simulink model "GolfSwingLogging"  (R2024b)
settings: Solver=VariableStepAuto  StartTime=0.0  StopTime=StopTime  MaxStep=0.001  RelTol=1e-3
PreLoadFcn:
  | cd(matlabdrive);
  | cd '2DModel';
PostLoadFcn:
  | %run SCRIPT_mdlWksGenerate.m;
  | mdlWks=get_param('GolfSwing','ModelWorkspace');
  | mdlWks.DataSource = 'MAT-File';
  | mdlWks.FileName = 'ModelInputs.mat';
  | mdlWks.reload;
model workspace: external: MAT-File ModelInputs.mat (data not in the file)
undefined symbols (not defined in the file or in its folder): GlobalGain, HipConstant, HipDampening, HipTimeGain, KillDampFinalValue, KillDampInitialValue, KillswitchFinalValue, KillswitchInitialValue, KillswitchStepTime, LElbowConstant, LElbowDampening, LElbowTimeGain, LScapConstant, LScapDampening, LScapPositionGain, LScapTimeGain, LShoulderConstant, LShoulderDampening, LShoulderTimeGain, LWristConstant, LWristDampening, LWristTimeGain, RElbowConstant, RElbowDampening, RElbowTimeGain, RScapConstant, RScapDampening, RScapPositionGain, RScapTimeGain, RShoulderConstant, RShoulderDampening, RShoulderTimeGain, RWristConstant, RWristDampening, RWristTimeGain, TorsoConstant, TorsoDampening, TorsoPositionGain, TorsoTimeGain, WristGain, X, Y, Z
libraries: nesl_utility x204, sm_lib x102, matrix_library x11, simulink_extras x2, simulink x1
(part 5 of 6)

== system GolfSwingLogging/Club/ButtGlobal ==
  Buttx : nesl_utility/PS-Simulink Converter  PhysicalDomain=network_engine_domain  SubClassName=ps_output  LeftPortType=input  RightPortType=output  PseudoPeriodic=off  Frequencies=[]  VectorFormat=1-D array  Unit=inherit  AffineConversion=off
  Butty : nesl_utility/PS-Simulink Converter  PhysicalDomain=network_engine_domain  SubClassName=ps_output  LeftPortType=input  RightPortType=output  PseudoPeriodic=off  Frequencies=[]  VectorFormat=1-D array  Unit=inherit  AffineConversion=off
  Buttz : nesl_utility/PS-Simulink Converter  PhysicalDomain=network_engine_domain  SubClassName=ps_output  LeftPortType=input  RightPortType=output  PseudoPeriodic=off  Frequencies=[]  VectorFormat=1-D array  Unit=inherit  AffineConversion=off
  Transform Sensor : sm_lib/Frames and Transforms/Transform Sensor  MeasurementFrame=World  RotationSequence=XYX  SenseAngle=off  SenseAxis=off  SenseQ=off  SenseR=off  SenseRotationSequence=off  SenseOmegaX=off  SenseOmegaY=off  SenseOmegaZ=off  SenseOmega=off  SenseQDot=off  SenseRDot=off  SenseRotationSequenceDot=off  SenseAlphaX=off  SenseAlphaY=off  SenseAlphaZ=off  SenseAlpha=off  SenseQDDot=off  SenseRDDot=off  SenseX=on  SenseY=on  SenseZ=on  SenseXYZ=off  SenseRad=off  SenseAzim=off  SenseDist=off  SenseInc=off  SenseXDot=off  SenseYDot=off  SenseZDot=off  SenseXYZDot=off  SenseRadDot=off  SenseAzimDot=off  SenseDistDot=off  SenseIncDot=off  SenseXDDot=off  SenseYDDot=off  SenseZDDot=off  SenseXYZDDot=off  SenseRadDDot=off  SenseAzimDDot=off  SenseDistDDot=off  SenseIncDDot=off
  Conn1 : PMIOPort  Side=Right
  Conn2 : PMIOPort  Port=2  Side=Left
  connections:
  Buttx/LConn1 -- Transform Sensor/RConn2
  Buttz/LConn1 -- Transform Sensor/RConn4
  Butty/LConn1 -- Transform Sensor/RConn3
  Transform Sensor/LConn1 -- Conn2/RConn1
  Transform Sensor/RConn1 -- Conn1/RConn1

== system GolfSwingLogging/Club/CHGlobal ==
  AoA Calculation : Subsystem
  CHS (m/s) : Subsystem
  CHSmph : Gain  Gain=2.23694
  CHvx : nesl_utility/PS-Simulink Converter  PhysicalDomain=network_engine_domain  SubClassName=ps_output  LeftPortType=input  RightPortType=output  PseudoPeriodic=off  Frequencies=[]  VectorFormat=1-D array  Unit=inherit  AffineConversion=off
  CHvy : nesl_utility/PS-Simulink Converter  PhysicalDomain=network_engine_domain  SubClassName=ps_output  LeftPortType=input  RightPortType=output  PseudoPeriodic=off  Frequencies=[]  VectorFormat=1-D array  Unit=inherit  AffineConversion=off
  CHvz : nesl_utility/PS-Simulink Converter  PhysicalDomain=network_engine_domain  SubClassName=ps_output  LeftPortType=input  RightPortType=output  PseudoPeriodic=off  Frequencies=[]  VectorFormat=1-D array  Unit=inherit  AffineConversion=off
  CHx : nesl_utility/PS-Simulink Converter  PhysicalDomain=network_engine_domain  SubClassName=ps_output  LeftPortType=input  RightPortType=output  PseudoPeriodic=off  Frequencies=[]  VectorFormat=1-D array  Unit=inherit  AffineConversion=off
  CHy : nesl_utility/PS-Simulink Converter  PhysicalDomain=network_engine_domain  SubClassName=ps_output  LeftPortType=input  RightPortType=output  PseudoPeriodic=off  Frequencies=[]  VectorFormat=1-D array  Unit=inherit  AffineConversion=off
  CHz : nesl_utility/PS-Simulink Converter  PhysicalDomain=network_engine_domain  SubClassName=ps_output  LeftPortType=input  RightPortType=output  PseudoPeriodic=off  Frequencies=[]  VectorFormat=1-D array  Unit=inherit  AffineConversion=off
  ClubheadPathUnitVector : Mux  Inputs=3
  Constant : Constant  Value=0
  Filtering Block : Subsystem  Commented=on
  MinMax Running Resettable : simulink/Math Operations/MinMax Running Resettable  Function=max  vinit=0.0
  Path Calculation : Subsystem
  Transform Sensor : sm_lib/Frames and Transforms/Transform Sensor  MeasurementFrame=World  RotationSequence=XYX  SenseAngle=off  SenseAxis=off  SenseQ=off  SenseR=off  SenseRotationSequence=off  SenseOmegaX=off  SenseOmegaY=off  SenseOmegaZ=off  SenseOmega=off  SenseQDot=off  SenseRDot=off  SenseRotationSequenceDot=off  SenseAlphaX=off  SenseAlphaY=off  SenseAlphaZ=off  SenseAlpha=off  SenseQDDot=off  SenseRDDot=off  SenseX=on  SenseY=on  SenseZ=on  SenseXYZ=off  SenseRad=off  SenseAzim=off  SenseDist=off  SenseInc=off  SenseXDot=on  SenseYDot=on  SenseZDot=on  SenseXYZDot=off  SenseRadDot=off  SenseAzimDot=off  SenseDistDot=off  SenseIncDot=off  SenseXDDot=off  SenseYDDot=off  SenseZDDot=off  SenseXYZDDot=off  SenseRadDDot=off  SenseAzimDDot=off  SenseDistDDot=off  SenseIncDDot=off
  UnitVectorX : Product  Inputs=*/
  UnitVectorY : Product  Inputs=*/
  UnitVectorZ : Product  Inputs=*/
  Clubhead : PMIOPort  Side=Right
  Global : PMIOPort  Port=2  Side=Left
  ClubPathUV : Outport
  CHSMPS : Outport  Port=2
  wires:
  CHvy/1 -> Path Calculation/1(Vy), AoA Calculation/2(Vy), UnitVectorY/1, CHS (m/s)/2(In2)  "CHvy"
  CHvx/1 -> AoA Calculation/1(Vx), Path Calculation/2(Vx), UnitVectorX/1, CHS (m/s)/1(In1)  "CHvx"
  CHvz/1 -> CHS (m/s)/3(In3), AoA Calculation/3(Vz), UnitVectorZ/1  "CHvz"
  UnitVectorZ/1 -> ClubheadPathUnitVector/3
  UnitVectorY/1 -> ClubheadPathUnitVector/2
  CHS (m/s)/1(ClubPathUV1) -> CHSMPS/1, CHSmph/1, UnitVectorZ/2, UnitVectorY/2, UnitVectorX/2  "CHSmpersec"
  UnitVectorX/1 -> ClubheadPathUnitVector/1
  ClubheadPathUnitVector/1 -> ClubPathUV/1  "ClubPathUV"
  CHSmph/1 -> MinMax Running Resettable/1, Filtering Block/1(CHS (mph))  "CHS (mph)"
  Constant/1 -> MinMax Running Resettable/2
  connections:
  CHx/LConn1 -- Transform Sensor/RConn2
  CHz/LConn1 -- Transform Sensor/RConn4
  CHvz/LConn1 -- Transform Sensor/RConn7
  CHy/LConn1 -- Transform Sensor/RConn3
  Transform Sensor/RConn5 -- CHvx/LConn1
  CHvy/LConn1 -- Transform Sensor/RConn6
  Transform Sensor/LConn1 -- Global/RConn1
  Transform Sensor/RConn1 -- Clubhead/RConn1

== system GolfSwingLogging/Club/Clubhead Air Resistance Calculator ==
  CHSmps : Inport
  ClubPathUV : Inport  Port=2
  Add : Sum  Inputs=+++
  Air Resistance : sm_lib/Forces and Torques/External Force and Torque  EnableForceX=off  EnableForceY=off  EnableForceZ=off  EnableForce=on  ForceResolutionFrame=World  EnableTorqueX=off  EnableTorqueY=off  EnableTorqueZ=off  EnableTorque=off  TorqueResolutionFrame=AttachedFrame
  Demux : Demux  Outputs=3
  Drag Function : MATLAB Function  TreatAsAtomicUnit=on
  Math Function : Math  Operator=square
  Math Function1 : Math  Operator=square
  Math Function2 : Math  Operator=square
  Matrix Multiply : Product
  Simulink-PS Converter : nesl_utility/Simulink-PS Converter  PhysicalDomain=network_engine_domain  SubClassName=ps_input  LeftPortType=input  RightPortType=output  PseudoPeriodic=off  Frequencies=[]  NoiseDistribution=none  NoiseParameters=[]  Unit=1  AffineConversion=off  FilteringAndDerivatives=provide  SimscapeFilterOrder=1  InputFilterTimeConstant=0.001  UdotUserProvided=0
  Sqrt : Sqrt
  FDrag : PMIOPort  Side=Right
  wires:
  ClubPathUV/1 -> Matrix Multiply/2
  Matrix Multiply/1 -> Demux/1, Simulink-PS Converter/1  "FDrag"
  CHSmps/1 -> Drag Function/1(u)
  Drag Function/1(FDrag) -> Matrix Multiply/1
  Add/1 -> Sqrt/1
  Math Function2/1 -> Add/3
  Math Function/1 -> Add/1
  Math Function1/1 -> Add/2
  Demux/2 -> Math Function1/1
  Demux/1 -> Math Function/1
  Demux/3 -> Math Function2/1
  connections:
  Air Resistance/RConn1 -- FDrag/RConn1
  Simulink-PS Converter/RConn1 -- Air Resistance/LConn1

== system GolfSwingLogging/Club/Flexible Beam Model ==
  Flexible Cylindrical Beam : sm_lib/Body Elements/Flexible Bodies/Beams/Flexible Cylindrical Beam  SectionType=Hollow  Radius=0.010  RadiusUnits=m  Thickness=0.0015  ThicknessUnits=m  Length=ShaftLength  LengthUnits=m  StiffnessAndInertiaType=CalculateFromGeometry  Density=500  DensityUnits=kg/m^3  ModuliType=YoungsPoissons  YoungsModulus=ShaftStiffness  YoungsModulusUnits=GPa  PoissonsRatio=0.33  ShearModulus=26  ShearModulusUnits=GPa  GeometricCentroid=[0 0]  GeometricCentroidUnits=m  BendingCentroid=[0 0]  BendingCentroidUnits=m  ShearCenter=[0 0]  ShearCenterUnits=m  AxialRigidity=1  AxialRigidityUnits=Pa*m^2  FlexuralRigidity=[1 1]  FlexuralRigidityUnits=Pa*m^4  CrossFlexuralRigidity=0  CrossFlexuralRigidityUnits=Pa*m^4  TorsionalRigidity=1  TorsionalRigidityUnits=Pa*m^4  CenterOfMass=[0 0]  CenterOfMassUnits=m  MassPerUnitLength=1  MassPerUnitLengthUnits=kg/m  MassMomentOfInertiaDensity=[1 1]  MassMomentOfInertiaDensityUnits=kg*m  MassProductOfInertiaDensity=0  MassProductOfInertiaDensityUnits=kg*m  DampingType=Proportional  ProportionalDampingAlpha=0  ProportionalDampingAlphaUnits=1/s  ProportionalDampingBeta=ShaftDampening  ProportionalDampingBetaUnits=s  UniformModalDampingRatio=0.01  NumElements=1  ReductionType=None  NumRetainedModes=1  GraphicType=FromGeometry  GraphicVisPropType=SimpleVisualProperties  GraphicDiffuseColor=[0.5 0.5 0.5]  GraphicOpacity=1.0  GraphicSpecularColor=[0.5 0.5 0.5 1.0]  GraphicAmbientColor=[0.15 0.15 0.15 1.0]  GraphicEmissiveColor=[0.0 0.0 0.0 1.0]  GraphicShininess=75  DoExposeZminFrame=on  DoExposeZmaxFrame=on  SerializedFrames=<Frames/>
  Rigid Transform : sm_lib/Frames and Transforms/Rigid Transform  RotationMethod=RotationSequence  FollAlignAxisA=+X  BaseAlignAxisA=+Y  FollAlignAxisB=+Y  BaseAlignAxisB=+Z  RotationStandardAxis=+Z  RotationAngle=0.0  RotationAngleUnits=deg  RotationArbitraryAxis=[0 0 1]  RotationSequenceAxes=FollowerAxes  RotationSequence=XYX  RotationSequenceAngles=[0 90 0]  RotationSequenceAnglesUnits=deg  RotationMatrix=[1 0 0; 0 1 0; 0 0 1]  Quaternion=[1 0 0 0]  TranslationMethod=None  TranslationCartesianOffset=[0 0 0]  TranslationCartesianOffsetUnits=m  TranslationStandardAxis=+Z  TranslationStandardOffset=0  TranslationStandardOffsetUnits=m  TranslationROffset=0  TranslationROffsetUnits=m  TranslationThetaOffset=0  TranslationThetaOffsetUnits=deg  TranslationZOffset=0  TranslationZOffsetUnits=m
  RH Grip : PMIOPort  Side=Left
  Clubhead : PMIOPort  Port=2  Side=Right
  connections:
  Rigid Transform/RConn1 -- Flexible Cylindrical Beam/LConn1
  RH Grip/RConn1 -- Rigid Transform/LConn1
  Flexible Cylindrical Beam/RConn1 -- Clubhead/RConn1

== system GolfSwingLogging/Club/Impact Model ==
  CHSmps : Inport
  ClubPathUV : Inport  Port=2
  Add1 : Sum
  Golf Ball Reaction Force : MATLAB Function  TreatAsAtomicUnit=on
  Golf Ball Rxn Force : sm_lib/Forces and Torques/External Force and Torque  EnableForceX=off  EnableForceY=off  EnableForceZ=off  EnableForce=on  ForceResolutionFrame=World  EnableTorqueX=off  EnableTorqueY=off  EnableTorqueZ=off  EnableTorque=off  TorqueResolutionFrame=AttachedFrame
  Matrix Multiply : Product
  Matrix Multiply1 : Product
  Simulink-PS Converter : nesl_utility/Simulink-PS Converter  PhysicalDomain=network_engine_domain  SubClassName=ps_input  LeftPortType=input  RightPortType=output  PseudoPeriodic=off  Frequencies=[]  NoiseDistribution=none  NoiseParameters=[]  Unit=1  AffineConversion=off  FilteringAndDerivatives=provide  SimscapeFilterOrder=1  InputFilterTimeConstant=0.001  UdotUserProvided=0
  Step : Step  Time=0.24  SampleTime=0
  Step1 : Step  Time=0.2405  After=-1  SampleTime=0
  FBRxn : PMIOPort  Side=Right
  wires:
  ClubPathUV/1 -> Matrix Multiply/2
  Matrix Multiply/1 -> Simulink-PS Converter/1  "FImpact"
  CHSmps/1 -> Golf Ball Reaction Force/1(u)
  Step1/1 -> Add1/2
  Step/1 -> Add1/1
  Add1/1 -> Matrix Multiply1/1
  Golf Ball Reaction Force/1(FImpact) -> Matrix Multiply1/2
  Matrix Multiply1/1 -> Matrix Multiply/1  "FImpactMag"
  connections:
  Golf Ball Rxn Force/RConn1 -- FBRxn/RConn1
  Simulink-PS Converter/RConn1 -- Golf Ball Rxn Force/LConn1

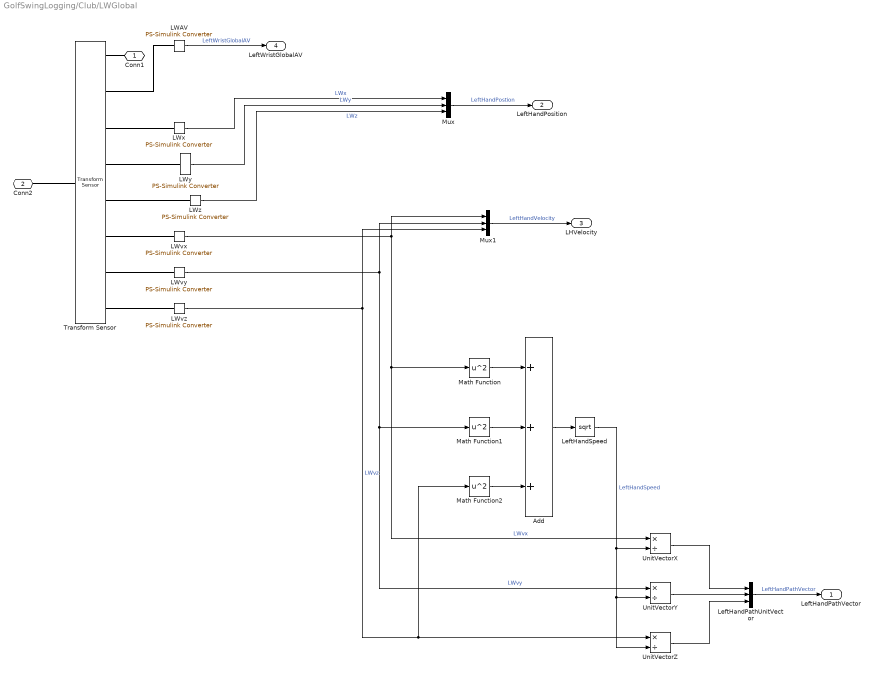
== system GolfSwingLogging/Club/LWGlobal ==
  Add : Sum  Inputs=+++
  LWAV : nesl_utility/PS-Simulink Converter  PhysicalDomain=network_engine_domain  SubClassName=ps_output  LeftPortType=input  RightPortType=output  PseudoPeriodic=off  Frequencies=[]  VectorFormat=1-D array  Unit=inherit  AffineConversion=off
  LWvx : nesl_utility/PS-Simulink Converter  PhysicalDomain=network_engine_domain  SubClassName=ps_output  LeftPortType=input  RightPortType=output  PseudoPeriodic=off  Frequencies=[]  VectorFormat=1-D array  Unit=inherit  AffineConversion=off
  LWvy : nesl_utility/PS-Simulink Converter  PhysicalDomain=network_engine_domain  SubClassName=ps_output  LeftPortType=input  RightPortType=output  PseudoPeriodic=off  Frequencies=[]  VectorFormat=1-D array  Unit=inherit  AffineConversion=off
  LWvz : nesl_utility/PS-Simulink Converter  PhysicalDomain=network_engine_domain  SubClassName=ps_output  LeftPortType=input  RightPortType=output  PseudoPeriodic=off  Frequencies=[]  VectorFormat=1-D array  Unit=inherit  AffineConversion=off
  LWx : nesl_utility/PS-Simulink Converter  PhysicalDomain=network_engine_domain  SubClassName=ps_output  LeftPortType=input  RightPortType=output  PseudoPeriodic=off  Frequencies=[]  VectorFormat=1-D array  Unit=inherit  AffineConversion=off
  LWy : nesl_utility/PS-Simulink Converter  PhysicalDomain=network_engine_domain  SubClassName=ps_output  LeftPortType=input  RightPortType=output  PseudoPeriodic=off  Frequencies=[]  VectorFormat=1-D array  Unit=inherit  AffineConversion=off
  LWz : nesl_utility/PS-Simulink Converter  PhysicalDomain=network_engine_domain  SubClassName=ps_output  LeftPortType=input  RightPortType=output  PseudoPeriodic=off  Frequencies=[]  VectorFormat=1-D array  Unit=inherit  AffineConversion=off
  LeftHandPathUnitVector : Mux  Inputs=3
  LeftHandSpeed : Sqrt
  Math Function : Math  Operator=square
  Math Function1 : Math  Operator=square
  Math Function2 : Math  Operator=square
  Mux : Mux  Inputs=3
  Mux1 : Mux  Inputs=3
  Transform Sensor : sm_lib/Frames and Transforms/Transform Sensor  MeasurementFrame=World  RotationSequence=XYX  SenseAngle=off  SenseAxis=off  SenseQ=off  SenseR=off  SenseRotationSequence=off  SenseOmegaX=off  SenseOmegaY=off  SenseOmegaZ=off  SenseOmega=on  SenseQDot=off  SenseRDot=off  SenseRotationSequenceDot=off  SenseAlphaX=off  SenseAlphaY=off  SenseAlphaZ=off  SenseAlpha=off  SenseQDDot=off  SenseRDDot=off  SenseX=on  SenseY=on  SenseZ=on  SenseXYZ=off  SenseRad=off  SenseAzim=off  SenseDist=off  SenseInc=off  SenseXDot=on  SenseYDot=on  SenseZDot=on  SenseXYZDot=off  SenseRadDot=off  SenseAzimDot=off  SenseDistDot=off  SenseIncDot=off  SenseXDDot=off  SenseYDDot=off  SenseZDDot=off  SenseXYZDDot=off  SenseRadDDot=off  SenseAzimDDot=off  SenseDistDDot=off  SenseIncDDot=off
  UnitVectorX : Product  Inputs=*/
  UnitVectorY : Product  Inputs=*/
  UnitVectorZ : Product  Inputs=*/
  Conn1 : PMIOPort  Side=Right
  Conn2 : PMIOPort  Port=2  Side=Left
  LeftHandPathVector : Outport
  LeftHandPosition : Outport  Port=2
  LHVelocity : Outport  Port=3
  LeftWristGlobalAV : Outport  Port=4
  wires:
  LWx/1 -> Mux/1  "LWx"
  LWy/1 -> Mux/2  "LWy"
  LWz/1 -> Mux/3  "LWz"
  UnitVectorZ/1 -> LeftHandPathUnitVector/3
  UnitVectorY/1 -> LeftHandPathUnitVector/2
  LeftHandPathUnitVector/1 -> LeftHandPathVector/1  "LeftHandPathVector"
  UnitVectorX/1 -> LeftHandPathUnitVector/1
  Add/1 -> LeftHandSpeed/1
  Math Function/1 -> Add/1
  Math Function1/1 -> Add/2
  Math Function2/1 -> Add/3
  LWvy/1 -> UnitVectorY/1, Math Function1/1, Mux1/2  "LWvy"
  LeftHandSpeed/1 -> UnitVectorX/2, UnitVectorY/2, UnitVectorZ/2  "LeftHandSpeed"
  LWvz/1 -> Mux1/3, Math Function2/1, UnitVectorZ/1  "LWvz"
  LWvx/1 -> Mux1/1, UnitVectorX/1, Math Function/1  "LWvx"
  Mux/1 -> LeftHandPosition/1  "LeftHandPostion"
  Mux1/1 -> LHVelocity/1  "LeftHandVelocity"
  LWAV/1 -> LeftWristGlobalAV/1  "LeftWristGlobalAV"
  connections:
  LWx/LConn1 -- Transform Sensor/RConn3
  LWz/LConn1 -- Transform Sensor/RConn5
  LWvz/LConn1 -- Transform Sensor/RConn8
  LWy/LConn1 -- Transform Sensor/RConn4
  LWvx/LConn1 -- Transform Sensor/RConn6
  LWvy/LConn1 -- Transform Sensor/RConn7
  Transform Sensor/LConn1 -- Conn2/RConn1
  Transform Sensor/RConn1 -- Conn1/RConn1
  LWAV/LConn1 -- Transform Sensor/RConn2

== system GolfSwingLogging/Club/MidpointGlobal ==
  Add : Sum  Inputs=+++
  Hand Speed (mph) : Gain  Gain=2.23694
  MPvx : nesl_utility/PS-Simulink Converter  PhysicalDomain=network_engine_domain  SubClassName=ps_output  LeftPortType=input  RightPortType=output  PseudoPeriodic=off  Frequencies=[]  VectorFormat=1-D array  Unit=inherit  AffineConversion=off
  MPvy : nesl_utility/PS-Simulink Converter  PhysicalDomain=network_engine_domain  SubClassName=ps_output  LeftPortType=input  RightPortType=output  PseudoPeriodic=off  Frequencies=[]  VectorFormat=1-D array  Unit=inherit  AffineConversion=off
  MPvz : nesl_utility/PS-Simulink Converter  PhysicalDomain=network_engine_domain  SubClassName=ps_output  LeftPortType=input  RightPortType=output  PseudoPeriodic=off  Frequencies=[]  VectorFormat=1-D array  Unit=inherit  AffineConversion=off
  MPx : nesl_utility/PS-Simulink Converter  PhysicalDomain=network_engine_domain  SubClassName=ps_output  LeftPortType=input  RightPortType=output  PseudoPeriodic=off  Frequencies=[]  VectorFormat=1-D array  Unit=inherit  AffineConversion=off
  MPy : nesl_utility/PS-Simulink Converter  PhysicalDomain=network_engine_domain  SubClassName=ps_output  LeftPortType=input  RightPortType=output  PseudoPeriodic=off  Frequencies=[]  VectorFormat=1-D array  Unit=inherit  AffineConversion=off
  MPz : nesl_utility/PS-Simulink Converter  PhysicalDomain=network_engine_domain  SubClassName=ps_output  LeftPortType=input  RightPortType=output  PseudoPeriodic=off  Frequencies=[]  VectorFormat=1-D array  Unit=inherit  AffineConversion=off
  Math Function : Math  Operator=square
  Math Function1 : Math  Operator=square
  Math Function2 : Math  Operator=square
  MidHandPathUnitVector : Mux  Inputs=3
  MidHandSpeed : Sqrt
  MidpointAV : nesl_utility/PS-Simulink Converter  PhysicalDomain=network_engine_domain  SubClassName=ps_output  LeftPortType=input  RightPortType=output  PseudoPeriodic=off  Frequencies=[]  VectorFormat=1-D array  Unit=inherit  AffineConversion=off
  Mux : Mux  Inputs=3
  Mux1 : Mux  Inputs=3
  Transform Sensor : sm_lib/Frames and Transforms/Transform Sensor  MeasurementFrame=World  RotationSequence=XYX  SenseAngle=off  SenseAxis=off  SenseQ=off  SenseR=off  SenseRotationSequence=off  SenseOmegaX=off  SenseOmegaY=off  SenseOmegaZ=off  SenseOmega=on  SenseQDot=off  SenseRDot=off  SenseRotationSequenceDot=off  SenseAlphaX=off  SenseAlphaY=off  SenseAlphaZ=off  SenseAlpha=off  SenseQDDot=off  SenseRDDot=off  SenseX=on  SenseY=on  SenseZ=on  SenseXYZ=off  SenseRad=off  SenseAzim=off  SenseDist=off  SenseInc=off  SenseXDot=on  SenseYDot=on  SenseZDot=on  SenseXYZDot=off  SenseRadDot=off  SenseAzimDot=off  SenseDistDot=off  SenseIncDot=off  SenseXDDot=off  SenseYDDot=off  SenseZDDot=off  SenseXYZDDot=off  SenseRadDDot=off  SenseAzimDDot=off  SenseDistDDot=off  SenseIncDDot=off
  UnitVectorX : Product  Inputs=*/
  UnitVectorY : Product  Inputs=*/
  UnitVectorZ : Product  Inputs=*/
  Conn1 : PMIOPort  Side=Right
  Conn2 : PMIOPort  Port=2  Side=Left
  HandPathVector : Outport
  MidHandPosition : Outport  Port=2
  MidHandVelocity : Outport  Port=3
  wires:
  Math Function1/1 -> Add/2
  MidHandSpeed/1 -> UnitVectorZ/2, UnitVectorY/2, UnitVectorX/2, Hand Speed (mph)/1  "MidHandSpeed"
  Math Function/1 -> Add/1
  Math Function2/1 -> Add/3
  Add/1 -> MidHandSpeed/1
  UnitVectorX/1 -> MidHandPathUnitVector/1
  UnitVectorY/1 -> MidHandPathUnitVector/2
  UnitVectorZ/1 -> MidHandPathUnitVector/3
  MidHandPathUnitVector/1 -> HandPathVector/1  "MPPathVector"
  MPy/1 -> Mux/2  "MPy"
  MPz/1 -> Mux/3  "MPz"
  Mux/1 -> MidHandPosition/1  "MidHandPosition"
  MPx/1 -> Mux/1  "MPx"
  MPvy/1 -> Math Function1/1, UnitVectorY/1, Mux1/2  "MPvy"
  MPvz/1 -> Mux1/3, UnitVectorZ/1, Math Function2/1  "MPvz"
  Mux1/1 -> MidHandVelocity/1  "MidHandVelocity"
  MPvx/1 -> Mux1/1, UnitVectorX/1, Math Function/1  "MPvx"
  connections:
  MPx/LConn1 -- Transform Sensor/RConn3
  MPz/LConn1 -- Transform Sensor/RConn5
  MPvz/LConn1 -- Transform Sensor/RConn8
  MPy/LConn1 -- Transform Sensor/RConn4
  MPvx/LConn1 -- Transform Sensor/RConn6
  MPvy/LConn1 -- Transform Sensor/RConn7
  Transform Sensor/LConn1 -- Conn2/RConn1
  Transform Sensor/RConn1 -- Conn1/RConn1
  MidpointAV/LConn1 -- Transform Sensor/RConn2

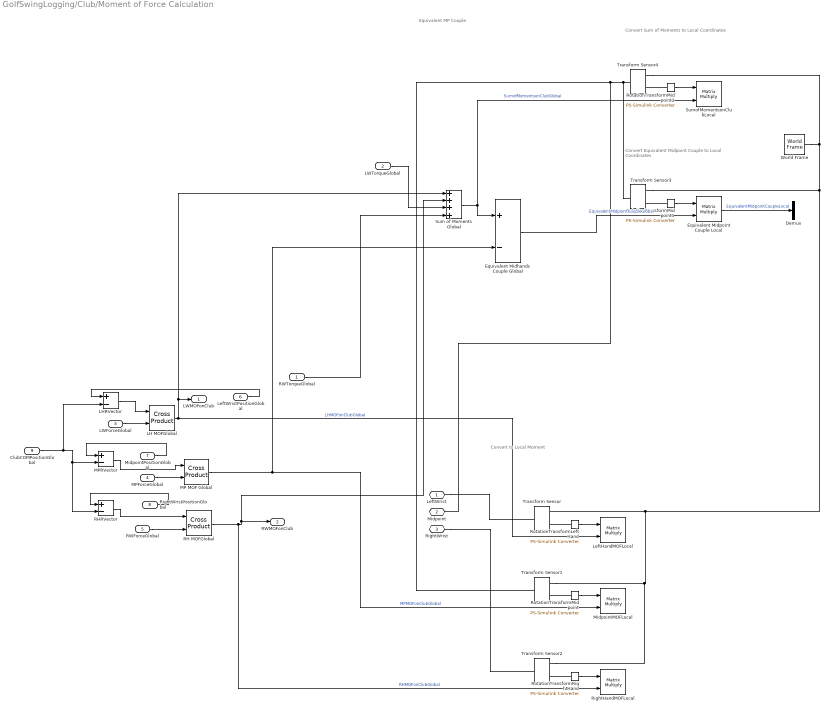
== system GolfSwingLogging/Club/Moment of Force Calculation ==
  note: Convert Sum of Moments to Local Coordinates
  note: Convert Equivalent Midpoint Couple to Local Coordinates
  note: Equivalent MP Couple
  note: Convert to Local Moment
  RWTorqueGlobal : Inport
  LWTorqueGlobal : Inport  Port=2
  LWForceGlobal : Inport  Port=3
  MPForceGlobal : Inport  Port=4
  RWForceGlobal : Inport  Port=5
  LeftWristPositionGlobal : Inport  Port=6
  MidpointPositionGlobal : Inport  Port=7
  RightWristPositionGlobal : Inport  Port=8
  ClubCOMPositionGlobal : Inport  Port=9
  Demux : Demux  Outputs=3
  Equivalent Midhands Couple Global : Sum  Inputs=+-
  Equivalent Midpoint Couple Local : Product  Multiplication=Matrix(*)
  LH MOFGlobal : matrix_library/Cross Product
  LHRVector : Sum  Inputs=+-
  LeftHandMOFLocal : Product  Multiplication=Matrix(*)
  MP MOF Global : matrix_library/Cross Product
  MPRVector : Sum  Inputs=+-
  MidpointMOFLocal : Product  Multiplication=Matrix(*)
  RH MOFGlobal : matrix_library/Cross Product
  RHRVector : Sum  Inputs=+-
  RightHandMOFLocal : Product  Multiplication=Matrix(*)
  RotationTransformLeftHand : nesl_utility/PS-Simulink Converter  PhysicalDomain=network_engine_domain  SubClassName=ps_output  LeftPortType=input  RightPortType=output  PseudoPeriodic=off  Frequencies=[]  VectorFormat=1-D array  Unit=inherit  AffineConversion=off
  RotationTransformMidpoint : nesl_utility/PS-Simulink Converter  PhysicalDomain=network_engine_domain  SubClassName=ps_output  LeftPortType=input  RightPortType=output  PseudoPeriodic=off  Frequencies=[]  VectorFormat=1-D array  Unit=inherit  AffineConversion=off
  RotationTransformMidpoint1 : nesl_utility/PS-Simulink Converter  PhysicalDomain=network_engine_domain  SubClassName=ps_output  LeftPortType=input  RightPortType=output  PseudoPeriodic=off  Frequencies=[]  VectorFormat=1-D array  Unit=inherit  AffineConversion=off
  RotationTransformMidpoint2 : nesl_utility/PS-Simulink Converter  PhysicalDomain=network_engine_domain  SubClassName=ps_output  LeftPortType=input  RightPortType=output  PseudoPeriodic=off  Frequencies=[]  VectorFormat=1-D array  Unit=inherit  AffineConversion=off
  RotationTransformRightHand : nesl_utility/PS-Simulink Converter  PhysicalDomain=network_engine_domain  SubClassName=ps_output  LeftPortType=input  RightPortType=output  PseudoPeriodic=off  Frequencies=[]  VectorFormat=1-D array  Unit=inherit  AffineConversion=off
  Sum of Moments Global : Sum  Inputs=++++
  SumofMomentsonClubLocal : Product  Multiplication=Matrix(*)
  Transform Sensor{,1..4} (5 alike) : sm_lib/Frames and Transforms/Transform Sensor  MeasurementFrame=World  RotationSequence=XYX  SenseAngle=off  SenseAxis=off  SenseQ=off  SenseR=on  SenseRotationSequence=off  SenseOmegaX=off  SenseOmegaY=off  SenseOmegaZ=off  SenseOmega=off  SenseQDot=off  SenseRDot=off  SenseRotationSequenceDot=off  SenseAlphaX=off  SenseAlphaY=off  SenseAlphaZ=off  SenseAlpha=off  SenseQDDot=off  SenseRDDot=off  SenseX=off  SenseY=off  SenseZ=off  SenseXYZ=off  SenseRad=off  SenseAzim=off  SenseDist=off  SenseInc=off  SenseXDot=off  SenseYDot=off  SenseZDot=off  SenseXYZDot=off  SenseRadDot=off  SenseAzimDot=off  SenseDistDot=off  SenseIncDot=off  SenseXDDot=off  SenseYDDot=off  SenseZDDot=off  SenseXYZDDot=off  SenseRadDDot=off  SenseAzimDDot=off  SenseDistDDot=off  SenseIncDDot=off
  World Frame : sm_lib/Frames and Transforms/World Frame
  LeftWrist : PMIOPort  Side=Left
  Midpoint : PMIOPort  Port=2  Side=Left
  RightWrist : PMIOPort  Port=3  Side=Left
  LWMOFonClub : Outport
  RWMOFonClub : Outport  Port=2
  wires:
  RHRVector/1 -> RH MOFGlobal/1
  LHRVector/1 -> LH MOFGlobal/1
  LWForceGlobal/1 -> LH MOFGlobal/2
  LeftWristPositionGlobal/1 -> LHRVector/1
  ClubCOMPositionGlobal/1 -> RHRVector/2, MPRVector/2, LHRVector/2
  MidpointPositionGlobal/1 -> MPRVector/1
  RightWristPositionGlobal/1 -> RHRVector/1
  LH MOFGlobal/1 -> LWMOFonClub/1, Sum of Moments Global/1, LeftHandMOFLocal/2  "LHMOFonClubGlobal"
  MP MOF Global/1 -> Equivalent Midhands Couple Global/2, MidpointMOFLocal/2  "MPMOFonClubGlobal"
  RH MOFGlobal/1 -> Sum of Moments Global/2, RWMOFonClub/1, RightHandMOFLocal/2  "RHMOFonClubGlobal"
  MPForceGlobal/1 -> MP MOF Global/2
  MPRVector/1 -> MP MOF Global/1
  RWForceGlobal/1 -> RH MOFGlobal/2
  RotationTransformRightHand/1 -> RightHandMOFLocal/1
  RotationTransformMidpoint/1 -> MidpointMOFLocal/1
  RotationTransformLeftHand/1 -> LeftHandMOFLocal/1
  Equivalent Midhands Couple Global/1 -> Equivalent Midpoint Couple Local/2  "EquivalentMidpointCoupleGlobal"
  LWTorqueGlobal/1 -> Sum of Moments Global/3
  RWTorqueGlobal/1 -> Sum of Moments Global/4
  Sum of Moments Global/1 -> SumofMomentsonClubLocal/2, Equivalent Midhands Couple Global/1  "SumofMomentsonClubGlobal"
  RotationTransformMidpoint1/1 -> Equivalent Midpoint Couple Local/1
  RotationTransformMidpoint2/1 -> SumofMomentsonClubLocal/1
  Equivalent Midpoint Couple Local/1 -> Demux/1  "EquivalentMidpointCoupleLocal"
  connections:
  RightWrist/RConn1 -- Transform Sensor2/LConn1
  LeftWrist/RConn1 -- Transform Sensor/LConn1
  RotationTransformRightHand/LConn1 -- Transform Sensor2/RConn2
  RotationTransformMidpoint/LConn1 -- Transform Sensor1/RConn2
  RotationTransformLeftHand/LConn1 -- Transform Sensor/RConn2
  World Frame/RConn1 -- Transform Sensor3/RConn1 -- Transform Sensor1/RConn1 -- Transform Sensor2/RConn1 -- Transform Sensor/RConn1 -- Transform Sensor4/RConn1
  RotationTransformMidpoint1/LConn1 -- Transform Sensor3/RConn2
  Midpoint/RConn1 -- Transform Sensor3/LConn1 -- Transform Sensor4/LConn1 -- Transform Sensor1/LConn1
  RotationTransformMidpoint2/LConn1 -- Transform Sensor4/RConn2

== system GolfSwingLogging/Club/RWGlobal ==
  Add : Sum  Inputs=+++
  Math Function : Math  Operator=square
  Math Function1 : Math  Operator=square
  Math Function2 : Math  Operator=square
  Mux : Mux  Inputs=3
  Mux1 : Mux  Inputs=3
  RWAV : nesl_utility/PS-Simulink Converter  PhysicalDomain=network_engine_domain  SubClassName=ps_output  LeftPortType=input  RightPortType=output  PseudoPeriodic=off  Frequencies=[]  VectorFormat=1-D array  Unit=inherit  AffineConversion=off
  RWvx : nesl_utility/PS-Simulink Converter  PhysicalDomain=network_engine_domain  SubClassName=ps_output  LeftPortType=input  RightPortType=output  PseudoPeriodic=off  Frequencies=[]  VectorFormat=1-D array  Unit=inherit  AffineConversion=off
  RWvy : nesl_utility/PS-Simulink Converter  PhysicalDomain=network_engine_domain  SubClassName=ps_output  LeftPortType=input  RightPortType=output  PseudoPeriodic=off  Frequencies=[]  VectorFormat=1-D array  Unit=inherit  AffineConversion=off
  RWvz : nesl_utility/PS-Simulink Converter  PhysicalDomain=network_engine_domain  SubClassName=ps_output  LeftPortType=input  RightPortType=output  PseudoPeriodic=off  Frequencies=[]  VectorFormat=1-D array  Unit=inherit  AffineConversion=off
  RWx : nesl_utility/PS-Simulink Converter  PhysicalDomain=network_engine_domain  SubClassName=ps_output  LeftPortType=input  RightPortType=output  PseudoPeriodic=off  Frequencies=[]  VectorFormat=1-D array  Unit=inherit  AffineConversion=off
  RWy : nesl_utility/PS-Simulink Converter  PhysicalDomain=network_engine_domain  SubClassName=ps_output  LeftPortType=input  RightPortType=output  PseudoPeriodic=off  Frequencies=[]  VectorFormat=1-D array  Unit=inherit  AffineConversion=off
  RWz : nesl_utility/PS-Simulink Converter  PhysicalDomain=network_engine_domain  SubClassName=ps_output  LeftPortType=input  RightPortType=output  PseudoPeriodic=off  Frequencies=[]  VectorFormat=1-D array  Unit=inherit  AffineConversion=off
  RightHandPathUnitVector : Mux  Inputs=3
  RightHandSpeed : Sqrt
  Transform Sensor : sm_lib/Frames and Transforms/Transform Sensor  MeasurementFrame=World  RotationSequence=XYX  SenseAngle=off  SenseAxis=off  SenseQ=off  SenseR=off  SenseRotationSequence=off  SenseOmegaX=off  SenseOmegaY=off  SenseOmegaZ=off  SenseOmega=on  SenseQDot=off  SenseRDot=off  SenseRotationSequenceDot=off  SenseAlphaX=off  SenseAlphaY=off  SenseAlphaZ=off  SenseAlpha=off  SenseQDDot=off  SenseRDDot=off  SenseX=on  SenseY=on  SenseZ=on  SenseXYZ=off  SenseRad=off  SenseAzim=off  SenseDist=off  SenseInc=off  SenseXDot=on  SenseYDot=on  SenseZDot=on  SenseXYZDot=off  SenseRadDot=off  SenseAzimDot=off  SenseDistDot=off  SenseIncDot=off  SenseXDDot=off  SenseYDDot=off  SenseZDDot=off  SenseXYZDDot=off  SenseRadDDot=off  SenseAzimDDot=off  SenseDistDDot=off  SenseIncDDot=off
  UnitVectorX : Product  Inputs=*/
  UnitVectorY : Product  Inputs=*/
  UnitVectorZ : Product  Inputs=*/
  Conn1 : PMIOPort  Side=Right
  Conn2 : PMIOPort  Port=2  Side=Left
  RightHandPathVector : Outport
  RightHandPosition : Outport  Port=2
  RHVelocity : Outport  Port=3
  RightWristGlobalAV : Outport  Port=4
  wires:
  RightHandSpeed/1 -> UnitVectorZ/2, UnitVectorY/2, UnitVectorX/2  "RightHandSpeed"
  Math Function/1 -> Add/1
  Add/1 -> RightHandSpeed/1
  Math Function2/1 -> Add/3
  Math Function1/1 -> Add/2
  UnitVectorX/1 -> RightHandPathUnitVector/1
  RightHandPathUnitVector/1 -> RightHandPathVector/1  "RightHandPathVector"
  UnitVectorZ/1 -> RightHandPathUnitVector/3
  UnitVectorY/1 -> RightHandPathUnitVector/2
  RWy/1 -> Mux/2  "RWy"
  RWz/1 -> Mux/3  "RWz"
  Mux/1 -> RightHandPosition/1  "RightHandPosition"
  RWx/1 -> Mux/1  "RWx"
  RWvz/1 -> Math Function2/1, Mux1/3, UnitVectorZ/1  "RWvz"
  RWvy/1 -> UnitVectorY/1, Math Function1/1, Mux1/2  "RWvy"
  Mux1/1 -> RHVelocity/1  "RightHandVelocity"
  RWvx/1 -> UnitVectorX/1, Mux1/1, Math Function/1  "RWvx"
  RWAV/1 -> RightWristGlobalAV/1  "RightWristGlobalAV"
  connections:
  Transform Sensor/LConn1 -- Conn2/RConn1
  Transform Sensor/RConn1 -- Conn1/RConn1
  RWx/LConn1 -- Transform Sensor/RConn3
  RWy/LConn1 -- Transform Sensor/RConn4
  RWz/LConn1 -- Transform Sensor/RConn5
  RWvx/LConn1 -- Transform Sensor/RConn6
  RWvy/LConn1 -- Transform Sensor/RConn7
  RWvz/LConn1 -- Transform Sensor/RConn8
  RWAV/LConn1 -- Transform Sensor/RConn2

== system GolfSwingLogging/Club/Rigid Shaft ==
  Rigid Shaft : sm_lib/Body Elements/Cylindrical Solid  CylinderRadius=0.01  CylinderRadiusUnits=m  CylinderLength=1  CylinderLengthUnits=m  ExportEntireGeometry=off  InertiaType=CalculateFromGeometry  BasedOnType=Mass  Density=500  DensityUnits=kg/m^3  Mass=0.0802566  MassUnits=kg  CenterOfMass=[0 0 0]  CenterOfMassUnits=m  MomentsOfInertia=[1 1 1]  MomentsOfInertiaUnits=kg*m^2  ProductsOfInertia=[0 0 0]  ProductsOfInertiaUnits=kg*m^2  GraphicType=FromGeometry  MarkerShape=Sphere  MarkerSize=10  GraphicVisPropType=SimpleVisualProperties  GraphicDiffuseColor=[0.5 0.5 0.5]  GraphicOpacity=1.0  GraphicSpecularColor=[0.5 0.5 0.5 1.0]  GraphicAmbientColor=[0.15 0.15 0.15 1.0]  GraphicEmissiveColor=[0.0 0.0 0.0 1.0]  GraphicShininess=75  DoExposeReferenceFrame=off  SerializedFrames=<Frames><Frame><Id>Frame1</Id><Value><Name>RHGripTOS</Name><Origin><Source>GeometricFeature</Source><FeatureName>top curve</FeatureName></Origin><PrimaryAxis><DefinedDirection>-X</DefinedDirection><Source>ReferenceFrame</Source><SourceDirection>+Z</SourceDirection><FeatureName></FeatureName></PrimaryAxis><SecondaryAxis><DefinedDirection>+Y</DefinedDirection><Source>ReferenceFrame</Source><SourceDirection>+X</SourceDirection><FeatureName></FeatureName></SecondaryAxis></Value></Frame><Frame><Id>Frame2</Id><Value><Name>ShaftS1</Name><Origin><Source>GeometricFeature</Source><FeatureName>bottom curve</FeatureName></Origin><PrimaryAxis><DefinedDirection>-X</DefinedDirection><Source>ReferenceFrame</Source><SourceDirection>+Z</SourceDirection><FeatureName></FeatureName></PrimaryAxis><SecondaryAxis><DefinedDirection>+Y</DefinedDirection><Source>ReferenceFrame</Source><SourceDirection>+X</SourceDirection><FeatureName></FeatureName></SecondaryAxis></Value></Frame></Frames>
  RH : PMIOPort  Side=Right
  Clubhead : PMIOPort  Port=2  Side=Right
  connections:
  RH/RConn1 -- Rigid Shaft/LConn1
  Clubhead/RConn1 -- Rigid Shaft/RConn1

== system GolfSwingLogging/Club/Zero Mass Reference Shaft ==
  CHSCalculation : Subsystem  Commented=on
  CHvx : nesl_utility/PS-Simulink Converter  Commented=on  PhysicalDomain=network_engine_domain  SubClassName=ps_output  LeftPortType=input  RightPortType=output  PseudoPeriodic=off  Frequencies=[]  VectorFormat=1-D array  Unit=inherit  AffineConversion=off
  CHvy : nesl_utility/PS-Simulink Converter  Commented=on  PhysicalDomain=network_engine_domain  SubClassName=ps_output  LeftPortType=input  RightPortType=output  PseudoPeriodic=off  Frequencies=[]  VectorFormat=1-D array  Unit=inherit  AffineConversion=off
  CHvz : nesl_utility/PS-Simulink Converter  Commented=on  PhysicalDomain=network_engine_domain  SubClassName=ps_output  LeftPortType=input  RightPortType=output  PseudoPeriodic=off  Frequencies=[]  VectorFormat=1-D array  Unit=inherit  AffineConversion=off
  CHx : nesl_utility/PS-Simulink Converter  Commented=on  PhysicalDomain=network_engine_domain  SubClassName=ps_output  LeftPortType=input  RightPortType=output  PseudoPeriodic=off  Frequencies=[]  VectorFormat=1-D array  Unit=inherit  AffineConversion=off
  CHy : nesl_utility/PS-Simulink Converter  Commented=on  PhysicalDomain=network_engine_domain  SubClassName=ps_output  LeftPortType=input  RightPortType=output  PseudoPeriodic=off  Frequencies=[]  VectorFormat=1-D array  Unit=inherit  AffineConversion=off
  CHz : nesl_utility/PS-Simulink Converter  Commented=on  PhysicalDomain=network_engine_domain  SubClassName=ps_output  LeftPortType=input  RightPortType=output  PseudoPeriodic=off  Frequencies=[]  VectorFormat=1-D array  Unit=inherit  AffineConversion=off
  ClubheadPathUnitVector : Mux  Commented=on  Inputs=3
  ShaftPhysicalConfig : Subsystem
  Transform Sensor : sm_lib/Frames and Transforms/Transform Sensor  Commented=on  MeasurementFrame=World  RotationSequence=XYX  SenseAngle=off  SenseAxis=off  SenseQ=off  SenseR=off  SenseRotationSequence=off  SenseOmegaX=off  SenseOmegaY=off  SenseOmegaZ=off  SenseOmega=off  SenseQDot=off  SenseRDot=off  SenseRotationSequenceDot=off  SenseAlphaX=off  SenseAlphaY=off  SenseAlphaZ=off  SenseAlpha=off  SenseQDDot=off  SenseRDDot=off  SenseX=on  SenseY=on  SenseZ=on  SenseXYZ=off  SenseRad=off  SenseAzim=off  SenseDist=off  SenseInc=off  SenseXDot=on  SenseYDot=on  SenseZDot=on  SenseXYZDot=off  SenseRadDot=off  SenseAzimDot=off  SenseDistDot=off  SenseIncDot=off  SenseXDDot=off  SenseYDDot=off  SenseZDDot=off  SenseXYZDDot=off  SenseRadDDot=off  SenseAzimDDot=off  SenseDistDDot=off  SenseIncDDot=off
  UnitVectorX : Product  Commented=on  Inputs=*/
  UnitVectorY : Product  Commented=on  Inputs=*/
  UnitVectorZ : Product  Commented=on  Inputs=*/
  RH : PMIOPort  Side=Right
  ConnGlobal : PMIOPort  Port=2  Side=Right
  wires:
  CHvz/1 -> CHSCalculation/3(In1), UnitVectorZ/1
  CHvy/1 -> CHSCalculation/2(In3), UnitVectorY/1
  UnitVectorY/1 -> ClubheadPathUnitVector/2
  UnitVectorZ/1 -> ClubheadPathUnitVector/3
  CHSCalculation/1(Out1) -> UnitVectorY/2, UnitVectorZ/2, UnitVectorX/2  "GhostCHS"
  UnitVectorX/1 -> ClubheadPathUnitVector/1
  CHvx/1 -> CHSCalculation/1(In2), UnitVectorX/1
  connections:
  ShaftPhysicalConfig/RConn1 -- RH/RConn1
  ConnGlobal/RConn1 -- Transform Sensor/LConn1
  ShaftPhysicalConfig/RConn2 -- Transform Sensor/RConn1
  CHy/LConn1 -- Transform Sensor/RConn3
  CHvy/LConn1 -- Transform Sensor/RConn6
  CHx/LConn1 -- Transform Sensor/RConn2
  CHz/LConn1 -- Transform Sensor/RConn4
  CHvz/LConn1 -- Transform Sensor/RConn7
  CHvx/LConn1 -- Transform Sensor/RConn5

== system GolfSwingLogging/Right Wrist Joint/RightWristRelease ==
  note: To operate the right wrist release you need to set the right wrist joint configuration to "Provided by input" and then put this step function on the input and give it a release time and then the right hand will let go at that point in time.
  RIght Wrist Release : Step  Commented=on  After=-1  SampleTime=0
  Simulink-PS Converter : nesl_utility/Simulink-PS Converter  Commented=on  PhysicalDomain=network_engine_domain  SubClassName=ps_input  LeftPortType=input  RightPortType=output  PseudoPeriodic=off  Frequencies=[]  NoiseDistribution=none  NoiseParameters=[]  Unit=1  AffineConversion=off  FilteringAndDerivatives=provide  SimscapeFilterOrder=1  InputFilterTimeConstant=0.001  UdotUserProvided=0
  output : PMIOPort  Side=Right
  wires:
  RIght Wrist Release/1 -> Simulink-PS Converter/1
  connections:
  Simulink-PS Converter/RConn1 -- output/RConn1

== system GolfSwingLogging/Club/CHGlobal/AoA Calculation ==
  Vx : Inport
  Vy : Inport  Port=2
  Vz : Inport  Port=3
  Add : Sum
  AoA : simulink_extras/Transformations/Radians to Degrees
  Divide : Product  Inputs=*/
  Run : Sqrt
  Square : Math  Operator=square
  Square1 : Math  Operator=square
  atan : Trigonometry  Operator=atan
  wires:
  Vy/1 -> Square1/1
  Square/1 -> Add/1
  Run/1 -> Divide/2
  Square1/1 -> Add/2
  Vz/1 -> Divide/1
  Divide/1 -> atan/1
  Add/1 -> Run/1
  Vx/1 -> Square/1
  atan/1 -> AoA/1

== system GolfSwingLogging/Club/CHGlobal/CHS (m//s) ==
  In1 : Inport
  In2 : Inport  Port=2
  In3 : Inport  Port=3
  Add : Sum  Inputs=+++
  Math Function : Math  Operator=square
  Math Function1 : Math  Operator=square
  Math Function2 : Math  Operator=square
  Sqrt : Sqrt
  ClubPathUV1 : Outport
  wires:
  Math Function2/1 -> Add/3
  In1/1 -> Math Function/1
  In2/1 -> Math Function1/1
  Math Function/1 -> Add/1
  Add/1 -> Sqrt/1
  In3/1 -> Math Function2/1
  Sqrt/1 -> ClubPathUV1/1
  Math Function1/1 -> Add/2

== system GolfSwingLogging/Club/CHGlobal/Filtering Block ==
  CHS (mph) : Inport
  MATLAB Function : MATLAB Function  Commented=on  TreatAsAtomicUnit=on
  wires:
  CHS (mph)/1 -> MATLAB Function/1(u)

== system GolfSwingLogging/Club/CHGlobal/Path Calculation ==
  Vy : Inport
  Vx : Inport  Port=2
  Constant : Constant  Value=-1
  Divide : Product  Inputs=*/
  Path : simulink_extras/Transformations/Radians to Degrees
  PathCalc : Trigonometry  Operator=atan
  Product : Product
  wires:
  Vy/1 -> Divide/1
  Divide/1 -> PathCalc/1
  PathCalc/1 -> Product/1
  Vx/1 -> Divide/2
  Product/1 -> Path/1
  Constant/1 -> Product/2

== system GolfSwingLogging/Club/Zero Mass Reference Shaft/CHSCalculation ==
  In2 : Inport
  In3 : Inport  Port=2
  In1 : Inport  Port=3
  Add : Sum  Inputs=+++
  Math Function : Math  Operator=square
  Math Function1 : Math  Operator=square
  Math Function2 : Math  Operator=square
  Sqrt : Sqrt
  Out1 : Outport
  wires:
  Math Function2/1 -> Add/3
  In1/1 -> Math Function/1
  In2/1 -> Math Function1/1
  Math Function/1 -> Add/1
  Add/1 -> Sqrt/1
  In3/1 -> Math Function2/1
  Sqrt/1 -> Out1/1
  Math Function1/1 -> Add/2

== system GolfSwingLogging/Club/Zero Mass Reference Shaft/ShaftPhysicalConfig ==
  GhostShaft : sm_lib/Body Elements/Cylindrical Solid  CylinderRadius=0.01  CylinderRadiusUnits=m  CylinderLength=1  CylinderLengthUnits=m  ExportEntireGeometry=off  InertiaType=CalculateFromGeometry  BasedOnType=Mass  Density=500  DensityUnits=kg/m^3  Mass=0  MassUnits=kg  CenterOfMass=[0 0 0]  CenterOfMassUnits=m  MomentsOfInertia=[1 1 1]  MomentsOfInertiaUnits=kg*m^2  ProductsOfInertia=[0 0 0]  ProductsOfInertiaUnits=kg*m^2  GraphicType=FromGeometry  MarkerShape=Sphere  MarkerSize=10  GraphicVisPropType=SimpleVisualProperties  GraphicDiffuseColor=[0.2 0.2 1.0]  GraphicOpacity=1.0  GraphicSpecularColor=[0.5 0.5 0.5 1.0]  GraphicAmbientColor=[0.15 0.15 0.15 1.0]  GraphicEmissiveColor=[0.0 0.0 0.0 1.0]  GraphicShininess=75  DoExposeReferenceFrame=off  SerializedFrames=<Frames><Frame><Id>Frame1</Id><Value><Name>RHGripTOS</Name><Origin><Source>GeometricFeature</Source><FeatureName>top curve</FeatureName></Origin><PrimaryAxis><DefinedDirection>-X</DefinedDirection><Source>ReferenceFrame</Source><SourceDirection>+Z</SourceDirection><FeatureName></FeatureName></PrimaryAxis><SecondaryAxis><DefinedDirection>+Y</DefinedDirection><Source>ReferenceFrame</Source><SourceDirection>+X</SourceDirection><FeatureName></FeatureName></SecondaryAxis></Value></Frame><Frame><Id>Frame2</Id><Value><Name>GhostClubhead</Name><Origin><Source>GeometricFeature</Source><FeatureName>bottom curve</FeatureName></Origin><PrimaryAxis><DefinedDirection>+Z</DefinedDirection><Source>ReferenceFrame</Source><SourceDirection>+Z</SourceDirection><FeatureName></FeatureName></PrimaryAxis><SecondaryAxis><DefinedDirection>+X</DefinedDirection><Source>ReferenceFrame</Source><SourceDirection>+X</SourceDirection><FeatureName></FeatureName></SecondaryAxis></Value></Frame></Frames>
  PS-Simulink Converter14 : nesl_utility/PS-Simulink Converter  PhysicalDomain=network_engine_domain  SubClassName=ps_output  LeftPortType=input  RightPortType=output  PseudoPeriodic=off  Frequencies=[]  VectorFormat=inherit  Unit=inherit  AffineConversion=off
  RH : PMIOPort  Side=Right
  RH1 : PMIOPort  Port=2  Side=Right
  connections:
  GhostShaft/LConn1 -- RH/RConn1
  RH1/RConn1 -- GhostShaft/RConn1

== matlab function GolfSwingLogging/RJM Inputs/Left Shoulder Input Torque ==
  data: Time input; LeftShoulderTimeGain input; JointTorqueLShoulder output; LeftShoulderConstant input; LeftShoulderVelocity input; LeftShoulderDamper input; Killswitch input; GlobalGain input; KillDamp input
function JointTorqueLShoulder = fcn(Time,LeftShoulderTimeGain,LeftShoulderConstant,LeftShoulderVelocity,LeftShoulderDamper,Killswitch,GlobalGain,KillDamp)
JointTorqueLShoulder = Killswitch*GlobalGain*(LeftShoulderTimeGain*Time+LeftShoulderConstant)-GlobalGain*KillDamp*(LeftShoulderVelocity*LeftShoulderDamper);

== matlab function GolfSwingLogging/RJM Inputs/Right Shoulder Input Torque ==
  data: Time input; RightShoulderTimeGain input; JointTorqueRShoulder output; RightShoulderConstant input; RightShoulderVelocity input; RightShoulderDamper input; Killswitch input; GlobalGain input; KillDamp input
function JointTorqueRShoulder = fcn(Time,RightShoulderTimeGain,RightShoulderConstant,RightShoulderVelocity,RightShoulderDamper,Killswitch,GlobalGain,KillDamp)
JointTorqueRShoulder = Killswitch*GlobalGain*(RightShoulderTimeGain*Time+RightShoulderConstant)-GlobalGain*KillDamp*RightShoulderVelocity*RightShoulderDamper;

== matlab function GolfSwingLogging/RJM Inputs/Left Wrist Input Torque ==
  data: Time input; LeftWristTimeGain input; JointTorqueLWrist output; LeftWristConstant input; LeftWristVelocity input; LeftWristDamper input; Killswitch input; GlobalGain input; KillDamp input; WristGain input
function JointTorqueLWrist = fcn(Time,LeftWristTimeGain,LeftWristConstant,LeftWristVelocity,LeftWristDamper,Killswitch,GlobalGain,KillDamp,WristGain)
JointTorqueLWrist = WristGain*(Killswitch*GlobalGain*(LeftWristTimeGain*Time+LeftWristConstant)-GlobalGain*KillDamp*LeftWristVelocity*LeftWristDamper);

== matlab function GolfSwingLogging/RJM Inputs/Right Wrist Input Torque ==
  data: Time input; RightWristTimeGain input; JointTorqueRWrist output; RightWristConstant input; RightWristVelocity input; RightWristDamper input; Killswitch input; GlobalGain input; KillDamp input; WristGain input
function JointTorqueRWrist = fcn(Time,RightWristTimeGain,RightWristConstant,RightWristVelocity,RightWristDamper,Killswitch,GlobalGain,KillDamp,WristGain)
JointTorqueRWrist = WristGain*(Killswitch*GlobalGain*(RightWristTimeGain*Time+RightWristConstant)-GlobalGain*KillDamp*RightWristVelocity*RightWristDamper);

== matlab function GolfSwingLogging/RJM Inputs/Left Elbow Input Torque ==
  data: Time input; LeftElbowTimeGain input; JointTorqueLElbow output; LeftElbowConstant input; LeftElbowVelocity input; LeftElbowDamper input; Killswitch input; GlobalGain input; KillDamp input
function JointTorqueLElbow = fcn(Time,LeftElbowTimeGain,LeftElbowConstant,LeftElbowVelocity,LeftElbowDamper,Killswitch,GlobalGain,KillDamp)
JointTorqueLElbow = Killswitch*GlobalGain*(LeftElbowTimeGain*Time+LeftElbowConstant)-GlobalGain*KillDamp*LeftElbowVelocity*LeftElbowDamper;

== matlab function GolfSwingLogging/RJM Inputs/Right Elbow Input Torque ==
  data: Time input; RightElbowTimeGain input; JointTorqueRElbow output; RightElbowConstant input; RightElbowVelocity input; RightElbowDamper input; Killswitch input; GlobalGain input; KillDamp input
function JointTorqueRElbow = fcn(Time,RightElbowTimeGain,RightElbowConstant,RightElbowVelocity,RightElbowDamper,Killswitch,GlobalGain,KillDamp)
JointTorqueRElbow = Killswitch*GlobalGain*(RightElbowTimeGain*Time+RightElbowConstant)-GlobalGain*KillDamp*(RightElbowVelocity*RightElbowDamper);

== matlab function GolfSwingLogging/Club/CHGlobal/Filtering Block/MATLAB Function ==
  data: u input; y output
function y = fcn(u)
% Need to figure out how to design a filter and use the filtfilt function
% as it is a zero phase shift filter.

% function y = fcn(u)
% 
% y = filtfilt();

== matlab function GolfSwingLogging/RJM Inputs/DeltaFunction ==
  data: Time input; WristGain input; LeftWristTimeGain input; JointTorqueDelta output; LeftWristConstant input; LeftWristVelocity input; LeftWristDamper input; Killswitch input; GlobalGain input; KillDamp input; RightWristTimeGain input; RightWristConstant input; RightWristVelocity input; RightWristDamper input; LeftElbowTimeGain input; LeftElbowConstant input; LeftElbowVelocity input; LeftElbowDamper input; RightElbowTimeGain input; RightElbowConstant input; RightElbowVelocity input; RightElbowDamper input; LeftShoulderTimeGain input; LeftShoulderConstant input; LeftShoulderVelocity input; LeftShoulderDamper input; RightShoulderTimeGain input; RightShoulderConstant input; RightShoulderVelocity input; RightShoulderDamper input
function JointTorqueDelta = fcn(Time,WristGain,LeftWristTimeGain,LeftWristConstant,LeftWristVelocity,LeftWristDamper,Killswitch,GlobalGain,KillDamp,RightWristTimeGain,RightWristConstant,RightWristVelocity,RightWristDamper,LeftElbowTimeGain,LeftElbowConstant,LeftElbowVelocity,LeftElbowDamper,RightElbowTimeGain,RightElbowConstant,RightElbowVelocity,RightElbowDamper,LeftShoulderTimeGain,LeftShoulderConstant,LeftShoulderVelocity,LeftShoulderDamper,RightShoulderTimeGain,RightShoulderConstant,RightShoulderVelocity,RightShoulderDamper)

% Turn off delta function:
JointTorqueDelta = 0;

% In order to make left wrist torque equal to zero, the delta needs to be
% set to the following function:
% JointTorqueDelta = -(WristGain*(Killswitch*GlobalGain*(LeftWristTimeGain*Time+LeftWristConstant)-GlobalGain*KillDamp*LeftWristVelocity*LeftWristDamper));

% In order to make right wrist torque equal to zero, the delta needs to be
% set to the following function:
% JointTorqueDelta = WristGain*(Killswitch*GlobalGain*(RightWristTimeGain*Time+RightWristConstant)-GlobalGain*KillDamp*RightWristVelocity*RightWristDamper);

% In order to make left elbow torque equal to zero, the delta needs to be
% set to the following function:
% JointTorqueDelta = -(Killswitch*GlobalGain*(LeftElbowTimeGain*Time+LeftElbowConstant)-GlobalGain*KillDamp*LeftElbowVelocity*LeftElbowDamper);

% In order to make right elbow torque equal to zero, the delta needs to be
% set to the following function:
% JointTorqueDelta = (Killswitch*GlobalGain*(RightElbowTimeGain*Time+RightElbowConstant)-GlobalGain*KillDamp*(RightElbowVelocity*RightElbowDamper));

% In order to make left shoulder torque equal to zero, the delta needs to be
% set to the following function:
% JointTorqueDelta = -(Killswitch*GlobalGain*(LeftShoulderTimeGain*Time+LeftShoulderConstant)-GlobalGain*KillDamp*(LeftShoulderVelocity*LeftShoulderDamper));

% In order to make right shoulder torque equal to zero, the delta needs to be
% set to the following function:
% JointTorqueDelta = (Killswitch*GlobalGain*(RightShoulderTimeGain*Time+RightShoulderConstant)-GlobalGain*KillDamp*RightShoulderVelocity*RightShoulderDamper);

% To split the wrist torque equally between the left and right wrist use
% the following fomula.
% JointTorqueDelta=-(WristGain*(Killswitch*GlobalGain*(LeftWristTimeGain*Time+LeftWristConstant)-GlobalGain*KillDamp*LeftWristVelocity*LeftWristDamper))+((WristGain*(Killswitch*GlobalGain*(LeftWristTimeGain*Time+LeftWristConstant)-GlobalGain*KillDamp*LeftWristVelocity*LeftWristDamper))+WristGain*(Killswitch*GlobalGain*(RightWristTimeGain*Time+RightWristConstant)-GlobalGain*KillDamp*RightWristVelocity*RightWristDamper))/2;

== matlab function GolfSwingLogging/MATLAB Function ==
  data: LateralConstant input; LateralForce output; LateralTimeGain input; Time input
function LateralForce = fcn(LateralConstant,LateralTimeGain,Time)

LateralForce = LateralConstant-Time*LateralTimeGain;
